simulink model "example"  (Simulink 7.8)
settings: Solver=ode45  StartTime=0.0  StopTime=inf  FixedStep=0.1  MaxStep=0.005  MinStep=0.005  RelTol=1e-12
libraries: model_lib x7
settings Model: Creator=mohammad  LastModifiedBy=mai03
settings DebuggingCC: SolverPrmCheckMsg=none  FcnCallInpInsideContextMsg=Use local settings  UnconnectedInputMsg=none  UnconnectedOutputMsg=none  UnconnectedLineMsg=none

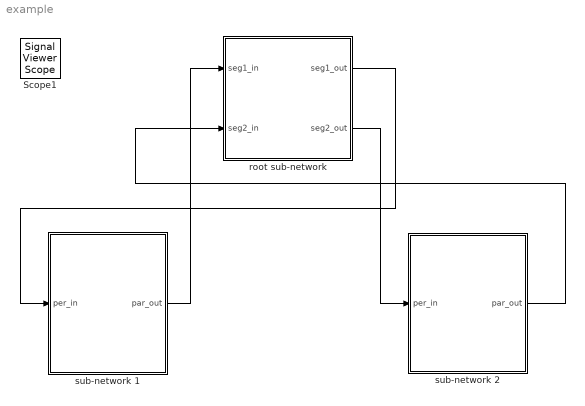
== system example ==
  root sub-network : Subsystem
  sub-network 1 : Subsystem
  sub-network 2 : Subsystem
  Scope1 : SignalViewerScope  IOType=viewer  RefreshTime=0.035000
  wires:
  sub-network 1/1(par_out) -> root sub-network/1(seg1_in)
  root sub-network/1(seg1_out) -> sub-network 1/1(per_in)
  root sub-network/2(seg2_out) -> sub-network 2/1(per_in)
  sub-network 2/1(par_out) -> root sub-network/2(seg2_in)

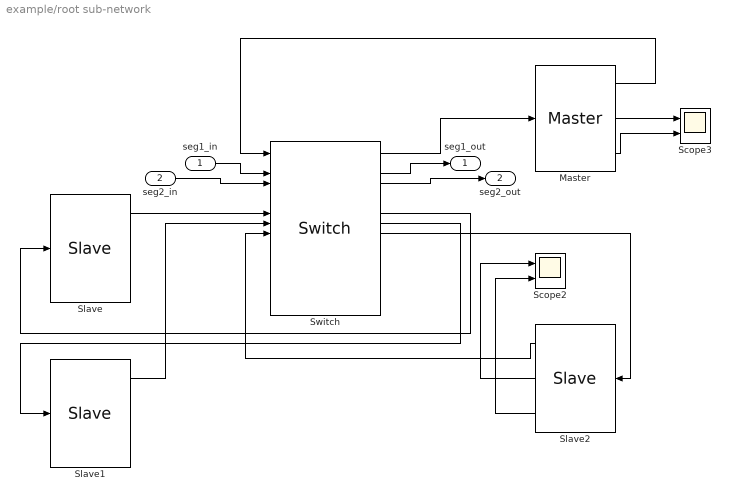
== system example/root sub-network ==
  seg1_in : Inport
  seg2_in : Inport  Port=2
  Master : model_lib/Master  Priority=2  master_number=1
  Scope2 : Scope  NumInputPorts=2
      settings: TimeRange=0.5  YMin=0~0  YMax=1~1
  Scope3 : Scope  NumInputPorts=2
      settings: TimeRange=0.5  YMin=0~0  YMax=1~1  SaveName=ScopeData3
  Slave : model_lib/Slave  Priority=3  slave_number=1
  Slave1 : model_lib/Slave  Priority=3  slave_number=2
  Slave2 : model_lib/Slave  Priority=3  slave_number=3
  Switch : model_lib/Switch  Priority=1  switch_number=1
  seg1_out : Outport
  seg2_out : Outport  Port=2
  wires:
  Master/2 -> Scope3/1
  Master/3 -> Scope3/2
  Switch/1 -> Master/1
  Master/1 -> Switch/1
  Slave/1 -> Switch/7
  Slave1/1 -> Switch/8
  Slave2/1 -> Switch/9
  Switch/7 -> Slave/1
  Switch/8 -> Slave1/1
  Switch/9 -> Slave2/1
  seg2_in/1 -> Switch/4
  seg1_in/1 -> Switch/3
  Switch/3 -> seg1_out/1
  Switch/4 -> seg2_out/1
  Slave2/2 -> Scope2/1
  Slave2/3 -> Scope2/2

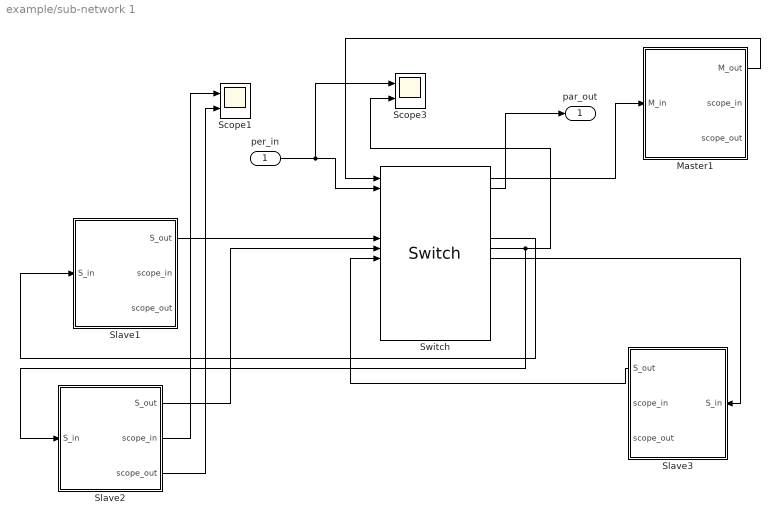
== system example/sub-network 1 ==
  per_in : Inport
  Master1 : Subsystem  Priority=1  mask{master_number=2}
      mask prompts: master_number "Master number"
  Scope1 : Scope  NumInputPorts=2
      settings: TimeRange=0.5  YMin=0~0  YMax=1~1  SaveName=ScopeData5
  Scope3 : Scope  NumInputPorts=2
      settings: TimeRange=0.5  YMin=0~0  YMax=1~1
  Slave1 : Subsystem  Priority=2  mask{slave_number=4}
      mask prompts: slave_number "Slave number"
  Slave2 : Subsystem  Priority=2  mask{slave_number=5}
      mask prompts: slave_number "Slave number"
  Slave3 : Subsystem  Priority=2  mask{slave_number=6}
      mask prompts: slave_number "Slave number"
  Switch : model_lib/Switch  switch_number=2
  par_out : Outport
  wires:
  Slave1/1(S_out) -> Switch/7
  Slave2/1(S_out) -> Switch/8
  Slave3/1(S_out) -> Switch/9
  Switch/7 -> Slave1/1(S_in)
  Switch/8 -> Slave2/1(S_in), Scope3/2
  Switch/9 -> Slave3/1(S_in)
  per_in/1 -> Switch/2, Scope3/1
  Switch/2 -> par_out/1
  Switch/1 -> Master1/1(M_in)
  Master1/1(M_out) -> Switch/1
  Slave2/2(scope_in) -> Scope1/1
  Slave2/3(scope_out) -> Scope1/2

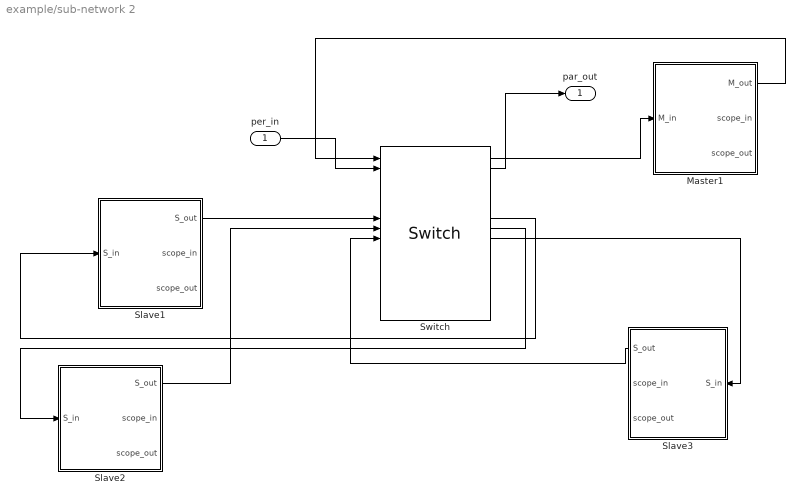
== system example/sub-network 2 ==
  per_in : Inport
  Master1 : Subsystem  Priority=1  mask{master_number=3}
      mask prompts: master_number "Master number"
  Slave1 : Subsystem  Priority=2  mask{slave_number=7}
      mask prompts: slave_number "Slave number"
  Slave2 : Subsystem  Priority=2  mask{slave_number=8}
      mask prompts: slave_number "Slave number"
  Slave3 : Subsystem  Priority=2  mask{slave_number=9}
      mask prompts: slave_number "Slave number"
  Switch : model_lib/Switch  switch_number=3
  par_out : Outport
  wires:
  Slave1/1(S_out) -> Switch/7
  Slave2/1(S_out) -> Switch/8
  Slave3/1(S_out) -> Switch/9
  Switch/7 -> Slave1/1(S_in)
  Switch/8 -> Slave2/1(S_in)
  Switch/9 -> Slave3/1(S_in)
  per_in/1 -> Switch/2
  Switch/2 -> par_out/1
  Switch/1 -> Master1/1(M_in)
  Master1/1(M_out) -> Switch/1

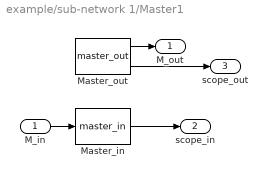
== system example/sub-network 1/Master1 ==
  M_in : Inport
  Master_in : M-S-Function  FunctionName=master_in
  Master_out : M-S-Function  FunctionName=master_out
  M_out : Outport
  scope_in : Outport  Port=2
  scope_out : Outport  Port=3
  wires:
  Master_out/1 -> M_out/1
  M_in/1 -> Master_in/1
  Master_in/1 -> scope_in/1
  Master_out/2 -> scope_out/1

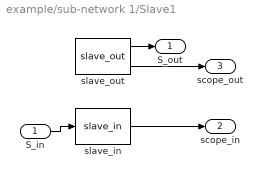
== system example/sub-network 1/Slave1 ==
  S_in : Inport
  slave_in : M-S-Function  FunctionName=slave_in
  slave_out : M-S-Function  FunctionName=slave_out
  S_out : Outport
  scope_in : Outport  Port=2
  scope_out : Outport  Port=3
  wires:
  slave_out/1 -> S_out/1
  S_in/1 -> slave_in/1
  slave_out/2 -> scope_out/1
  slave_in/1 -> scope_in/1

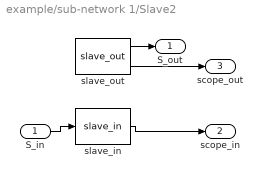
== system example/sub-network 1/Slave2 ==
  S_in : Inport
  slave_in : M-S-Function  FunctionName=slave_in
  slave_out : M-S-Function  FunctionName=slave_out
  S_out : Outport
  scope_in : Outport  Port=2
  scope_out : Outport  Port=3
  wires:
  slave_out/1 -> S_out/1
  S_in/1 -> slave_in/1
  slave_out/2 -> scope_out/1
  slave_in/1 -> scope_in/1

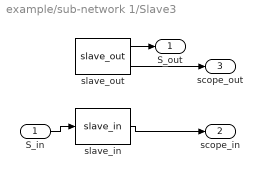
== system example/sub-network 1/Slave3 ==
  S_in : Inport
  slave_in : M-S-Function  FunctionName=slave_in
  slave_out : M-S-Function  FunctionName=slave_out
  S_out : Outport
  scope_in : Outport  Port=2
  scope_out : Outport  Port=3
  wires:
  slave_out/1 -> S_out/1
  S_in/1 -> slave_in/1
  slave_out/2 -> scope_out/1
  slave_in/1 -> scope_in/1

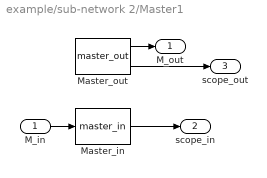
== system example/sub-network 2/Master1 ==
  M_in : Inport
  Master_in : M-S-Function  FunctionName=master_in
  Master_out : M-S-Function  FunctionName=master_out
  M_out : Outport
  scope_in : Outport  Port=2
  scope_out : Outport  Port=3
  wires:
  Master_out/1 -> M_out/1
  M_in/1 -> Master_in/1
  Master_in/1 -> scope_in/1
  Master_out/2 -> scope_out/1

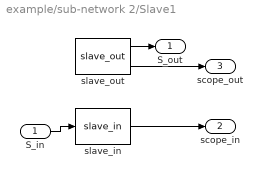
== system example/sub-network 2/Slave1 ==
  S_in : Inport
  slave_in : M-S-Function  FunctionName=slave_in
  slave_out : M-S-Function  FunctionName=slave_out
  S_out : Outport
  scope_in : Outport  Port=2
  scope_out : Outport  Port=3
  wires:
  slave_out/1 -> S_out/1
  S_in/1 -> slave_in/1
  slave_out/2 -> scope_out/1
  slave_in/1 -> scope_in/1

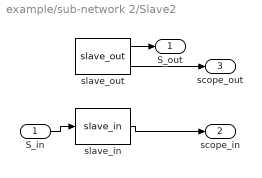
== system example/sub-network 2/Slave2 ==
  S_in : Inport
  slave_in : M-S-Function  FunctionName=slave_in
  slave_out : M-S-Function  FunctionName=slave_out
  S_out : Outport
  scope_in : Outport  Port=2
  scope_out : Outport  Port=3
  wires:
  slave_out/1 -> S_out/1
  S_in/1 -> slave_in/1
  slave_out/2 -> scope_out/1
  slave_in/1 -> scope_in/1

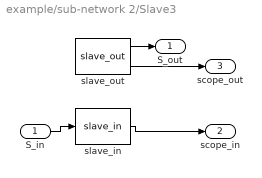
== system example/sub-network 2/Slave3 ==
  S_in : Inport
  slave_in : M-S-Function  FunctionName=slave_in
  slave_out : M-S-Function  FunctionName=slave_out
  S_out : Outport
  scope_in : Outport  Port=2
  scope_out : Outport  Port=3
  wires:
  slave_out/1 -> S_out/1
  S_in/1 -> slave_in/1
  slave_out/2 -> scope_out/1
  slave_in/1 -> scope_in/1
